simulink model "openloop_thyristor_w_control_initial_version"  (R2019b)
settings: Solver=VariableStepAuto  StartTime=0.0  StopTime=10  RelTol=1e-3
undefined symbols (not defined in the file): D1, lagging, pulse, sigbuilder_block
libraries: powerlib x20, powerlib_meascontrol x4, simulink x3
settings Model: Creator=82309  LastModifiedBy=82309
settings SolverCC: ZeroCrossAlgorithm=Adaptive
settings DebuggingCC: IgnoredZcDiagnostic=none

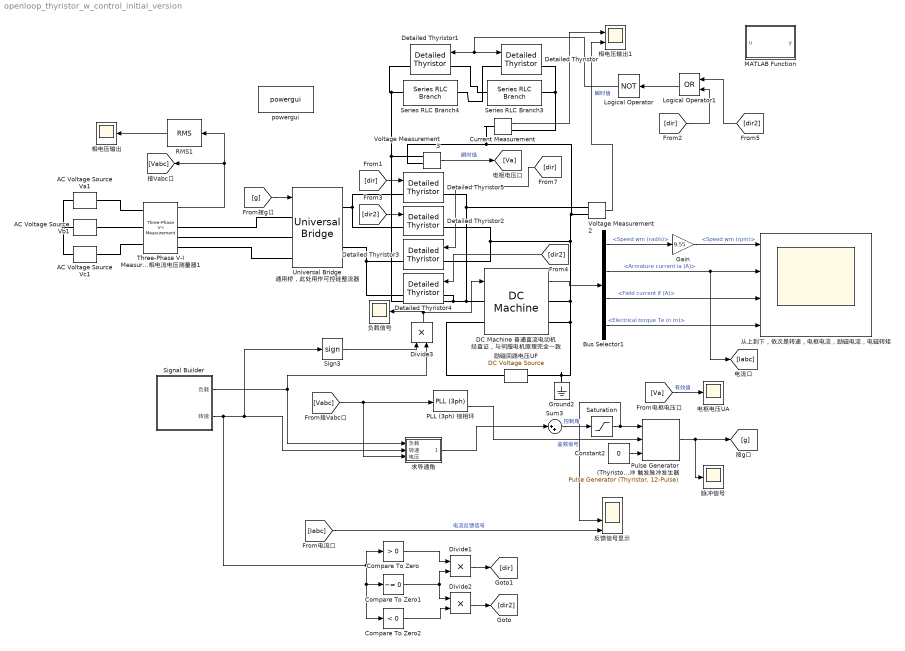
== system openloop_thyristor_w_control_initial_version ==
  AC Voltage Source Va1 : powerlib/Electrical Sources/AC Voltage Source  Amplitude=200  Phase=0  Frequency=60  SampleTime=0  Measurements=None  BusType=swing  Pref=10e3  Qref=0  Qmin=-inf  Qmax=+inf
      settings: SourceProductName=Simscape Electrical
  AC Voltage Source Vb1 : powerlib/Electrical Sources/AC Voltage Source  Amplitude=200  Phase=-120  Frequency=60  SampleTime=0  Measurements=None  BusType=swing  Pref=10e3  Qref=0  Qmin=-inf  Qmax=+inf
      settings: SourceProductName=Simscape Electrical
  AC Voltage Source Vc1 : powerlib/Electrical Sources/AC Voltage Source  Amplitude=200  Phase=-240  Frequency=60  SampleTime=0  Measurements=None  BusType=swing  Pref=10e3  Qref=0  Qmin=-inf  Qmax=+inf
      settings: SourceProductName=Simscape Electrical
  Bus Selector1 : BusSelector  OutputSignals=Speed wm (rad/s),Armature current ia (A),Field current if (A),Electrical torque Te (n m)
  Compare To Zero : simulink/Logic and Bit Operations/Compare To Zero  relop=>  OutDataTypeStr=boolean
  Compare To Zero1 : simulink/Logic and Bit Operations/Compare To Zero  relop=~=  OutDataTypeStr=boolean
  Compare To Zero2 : simulink/Logic and Bit Operations/Compare To Zero  relop=<  OutDataTypeStr=boolean
  Constant2 : Constant  Value=0
  Current Measurement : powerlib/Measurements/Current Measurement  PhasorSimulation=off  OutputType=Complex  PSBequivalent=0
      settings: SourceProductName=Simscape Electrical
  DC Machine 普通直流电动机 经查证，与伺服电机原理完全一致 : powerlib/Machines/DC Machine  PresetModel=01: 5HP 240V 1750RPM Field:300V  MechanicalLoad=Torque TL  FieldType=Wound  ShowDetailedParameters=on  MeasurementBus=off  RLa=[2.581 0.028]  RLf=[281.3 156]  Laf=0.9483  MachineConstant=Torque constant (N.m/A)  Ke=1.8  Kt=1.8  J=0.02215  Bm=0.002953  Tf=0.5161  w0=1  Ifinit=1  TsPowergui=0  TsBlock=-1
      settings: SourceProductName=Simscape Electrical
  Detailed Thyristor : powerlib/Power Electronics/Detailed Thyristor  Ron=0.001  Lon=1e-3  Vf=0.8  IL=0.1  Tq=100e-6  IC=0  Rs=inf  Cs=250e-9  Measurements=on
      settings: SourceProductName=Simscape Electrical  SourceProductBaseCode=PS
  Detailed Thyristor1 : powerlib/Power Electronics/Detailed Thyristor  Ron=0.001  Lon=1e-3  Vf=0.8  IL=0.1  Tq=100e-6  IC=0  Rs=inf  Cs=250e-9  Measurements=on
      settings: SourceProductName=Simscape Electrical  SourceProductBaseCode=PS
  Detailed Thyristor{2..5} (4 alike) : powerlib/Power Electronics/Detailed Thyristor  Ron=0.001  Lon=1e-3  Vf=0.8  IL=0.1  Tq=100e-6  IC=0  Rs=500  Cs=250e-9  Measurements=on
      settings: SourceProductName=Simscape Electrical  SourceProductBaseCode=PS
  Divide1 : Product  Inputs=**
  Divide2 : Product  Inputs=**
  Divide3 : Product  Inputs=**
  Gain : Gain  Gain=9.55
  Ground2 : powerlib/Elements/Ground  LConnTagsString=a
      settings: SourceProductName=Simscape Electrical
  Logical Operator : Logic  Operator=NOT  AllPortsSameDT=off  OutDataTypeStr=boolean
  Logical Operator1 : Logic  Operator=OR  AllPortsSameDT=off  OutDataTypeStr=boolean
  MATLAB Function : MATLAB Function  TreatAsAtomicUnit=on
  PLL (3ph) 锁相环 : powerlib_meascontrol/PLL/PLL (3ph)  Fmin=48  Par_Init=[0, 50]  ParK=[180, 3200, 1]  TcD=1e-4  MaxRateChangeFreq=12  FilterCutOffFreq=25  Ts=0  AGC=on
      settings: SourceProductName=Simscape Electrical
  "Pulse Generator (Thyristor, 6-Pulse) 六脉冲 触发脉冲发生器" : powerlib_meascontrol/Pulse & Signal Generators/Pulse Generator (Thyristor, 12-Pulse)  GenType=6-pulse  Delta=D1 (lagging)  pwidth=10  Double_Pulse=on  Ts=0
      settings: SourceProductName=Simscape Electrical  SourceProductBaseCode=PS
  RMS1 : powerlib_meascontrol/Measurements/RMS  TrueRMS=on  Freq=60  RMSInit=0  Ts=0
      settings: SourceProductName=Simscape Electrical
  Saturation : Saturate  UpperLimit=180  LowerLimit=0
  Series RLC Branch3 : powerlib/Elements/Series RLC Branch  LConnTagsString=__new0  RConnTagsString=__new0  BranchType=R  Resistance=1  Inductance=0.01  SetiL0=off  InitialCurrent=0  Capacitance=1e-6  Setx0=off  InitialVoltage=0  Measurements=None
      settings: SourceProductName=Simscape Electrical
  Series RLC Branch4 : powerlib/Elements/Series RLC Branch  LConnTagsString=__new0  RConnTagsString=__new0  BranchType=R  Resistance=1  Inductance=0.01  SetiL0=off  InitialCurrent=0  Capacitance=1e-6  Setx0=off  InitialVoltage=0  Measurements=None
      settings: SourceProductName=Simscape Electrical
  Sign3 : Signum
  Signal Builder : Subsystem  Tag=STV Subsys  LoadFcn=sigbuilder_block('load',[481.8 72 550.8 363.6 ]);  StartFcn=sigbuilder_block('start');  StopFcn=sigbuilder_block('stop');  ClipboardFcn=sigbuilder_block('clipboard');  mask(Sigbuilder block){tuvar=[0:10]}
      mask help: Sigbuilder GUI
      mask init:
      | if ~strcmp(get_param(bdroot(gcbh),'SimulationStatus'),'stopped') tuvar = sigbuilder_block('maskInit'); end
      settings: CopyFcn=sigbuilder_block('copy');  DeleteFcn=sigbuilder_block('delete');  ModelCloseFcn=sigbuilder_block('modelClose');  PreSaveFcn=sigbuilder_block('preSave');  PauseFcn=sigbuilder_block('pause')  ContinueFcn=sigbuilder_block('continue')  NameChangeFcn=sigbuilder_block('namechange');  OpenFcn=sigbuilder_block('open',[-27 31.8 550.8 363.6 ]);  CloseFcn=sigbuilder_block('close');
      mask Display: plot(0, 0, 100, 100,[2, 2, 32, 32, 2], [68, 8, 8, 68, 68],[32, 2], [38, 38], [32, 19, 2],[53, 60, 44], [32, 17, 17, 2],[16, 16, 31, 31]);txt = getActiveGroup(gcbh);text(2, 100, txt,'verticalAlignment', 'top');
  Sum3 : Sum  Inputs=|++
  Three-Phase V-I Measurement 三相电流电压测量器1 : powerlib/Measurements/Three-Phase V-I Measurement  VoltageMeasurement=phase-to-ground  SetLabelV=off  LabelV=Vabc  Vpu=off  VpuLL=off  CurrentMeasurement=yes  SetLabelI=off  LabelI=Iabc  Ipu=off  Pbase=100e6  Vbase=500e3  OutputType=Complex  PhasorSimulation=off  PSBequivalent=0
      settings: SourceProductName=Simscape Electrical
  Universal Bridge 通用桥，此处用作可控硅整流器 : powerlib/Power Electronics/Universal Bridge  Arms=3  SnubberResistance=1e5  SnubberCapacitance=inf  Device=Thyristors  Ron=1e-3  Lon=0  ForwardVoltages="[  0  0  ]"  ForwardVoltage=0  GTOparameters=[ 10e-6 , 20e-6 ]  IGBTparameters=[ 1e-6 , 2e-6 ]  Measurements=None  Measurements_2=None  converterType=Rectifier
      settings: SourceProductName=Simscape Electrical
  Voltage Measurement2 : powerlib/Measurements/Voltage Measurement  PhasorSimulation=off  OutputType=Complex  PSBequivalent=0
      settings: SourceProductName=Simscape Electrical
  Voltage Measurement3 : powerlib/Measurements/Voltage Measurement  PhasorSimulation=off  OutputType=Complex  PSBequivalent=0
      settings: SourceProductName=Simscape Electrical
  powergui : powerlib/powergui  Priority=1  SimulationMode=Continuous  SampleTime=50e-6  frequency=60  Iterations=50  frequencyindice=60  Pbase=100e6  ErrMax=1e-4  UnitsV=kV  UnitsW=MW  buscounter=0  FunctionMessages=off  echomessages=off  EnableUseOfTLC=off  CurrentSourceSwitches=off  DisableSnubberDevices=off  DisableRonSwitches=off  DisableVfSwitches=off  DisplayEquations=off  AutomaticDiscreteSolvers=off  SolverType=Tustin/Backward Euler (TBE)  Interpol=off  ExternalGateDelay=off  methode=off  Ts=100  x0status=blocks  SPID=on  SwTol=0  HookPort=off  NonlinearTolerance=1e-4  nMaxIteration=100  ContinueOnMaxIteration=off  RestoreLinks=warning  ResistiveCurrentMeasurement=off  Frange=[0:2:500]  Ylog=off  Xlog=on  ShowGrid=off  save=off  variable=ZData  structure=0  ZoomFFT=off  StartTime=0.0  cycles=1  DisplayStyle=1  fundamental=60  FreqAxis=off  MaxFrequency=1000  frequencyindicesteady=1  RmsSteady=1  display=off
      settings: SourceProductName=Simscape Electrical
  从上到下，依次是转速，电枢电流，励磁电流，电磁转矩 : Scope  NumInputPorts=4
  励磁回路电压UF : powerlib/Electrical Sources/DC Voltage Source  Amplitude=300  Measurements=None
      settings: SourceProductName=Simscape Electrical
  反馈信号显示 : Scope  NumInputPorts=4
  求导通角 : Subsystem
  电枢电压UA : Scope
  相电压输出 : Scope
  相电压输出1 : Scope  NumInputPorts=2
  脉冲信号 : Scope
  负载信号 : Scope
  wires:
  Bus Selector1/1 -> Gain/1  "<Speed wm (rad/s)>"
  Bus Selector1/3 -> 从上到下，依次是转速，电枢电流，励磁电流，电磁转矩/3  "<Field current if (A)>"
  "Pulse Generator (Thyristor, 6-Pulse) 六脉冲 触发脉冲发生器"/1 -> [g], 脉冲信号/1
  Three-Phase V-I Measurement 三相电流电压测量器1/1 -> RMS1/1, [Vabc]
  DC Machine 普通直流电动机 经查证，与伺服电机原理完全一致/1 -> Bus Selector1/1
  Constant2/1 -> "Pulse Generator (Thyristor, 6-Pulse) 六脉冲 触发脉冲发生器"/3
  [g] -> Universal Bridge 通用桥，此处用作可控硅整流器/1
  Bus Selector1/2 -> [Iabc], 从上到下，依次是转速，电枢电流，励磁电流，电磁转矩/2  "<Armature current ia (A)>"
  Gain/1 -> 从上到下，依次是转速，电枢电流，励磁电流，电磁转矩/1  "<Speed wm (rpm)>"
  Bus Selector1/4 -> 从上到下，依次是转速，电枢电流，励磁电流，电磁转矩/4  "<Electrical torque Te (n m)>"
  PLL (3ph) 锁相环/2 -> "Pulse Generator (Thyristor, 6-Pulse) 六脉冲 触发脉冲发生器"/2  "鉴频信号"
  [Vabc] -> PLL (3ph) 锁相环/1, 求导通角/3(电压)
  RMS1/1 -> 相电压输出/1
  Voltage Measurement3/1 -> [Va]  "瞬时值"
  Signal Builder/1(负载) -> 求导通角/1(负载), Divide3/2
  Logical Operator1/1 -> Logical Operator/1
  [Va] -> 电枢电压UA/1  "有效值"
  [Iabc] -> 反馈信号显示/4  "电流反馈信号"
  Saturation/1 -> "Pulse Generator (Thyristor, 6-Pulse) 六脉冲 触发脉冲发生器"/1, 反馈信号显示/3
  Sum3/1 -> Saturation/1  "控制角"
  求导通角/1(Out1) -> Sum3/1
  Voltage Measurement2/1 -> 相电压输出1/2  "瞬时值"
  Divide1/1 -> [dir]
  Compare To Zero/1 -> Divide1/1
  Compare To Zero1/1 -> Divide2/1, Divide1/2
  Compare To Zero2/1 -> Divide2/2
  Divide2/1 -> [dir2]
  [dir] -> Logical Operator1/2
  [dir2] -> Logical Operator1/1
  Logical Operator/1 -> Detailed Thyristor1/1, Detailed Thyristor/1
  Current Measurement/1 -> 相电压输出1/1
  [dir2] -> Detailed Thyristor2/1
  [dir] -> Detailed Thyristor5/1
  [dir2] -> Detailed Thyristor4/1
  [dir] -> Detailed Thyristor3/1
  Sign3/1 -> Divide3/1
  Divide3/1 -> DC Machine 普通直流电动机 经查证，与伺服电机原理完全一致/1, 负载信号/1
  Signal Builder/2(转速) -> Compare To Zero2/1, Compare To Zero1/1, Compare To Zero/1, Sign3/1, 求导通角/2(转速)
  connections:
  励磁回路电压UF/RConn1 -- DC Machine 普通直流电动机 经查证，与伺服电机原理完全一致/LConn2
  Three-Phase V-I Measurement 三相电流电压测量器1/RConn1 -- Universal Bridge 通用桥，此处用作可控硅整流器/LConn1
  Universal Bridge 通用桥，此处用作可控硅整流器/LConn2 -- Three-Phase V-I Measurement 三相电流电压测量器1/RConn2
  Three-Phase V-I Measurement 三相电流电压测量器1/RConn3 -- Universal Bridge 通用桥，此处用作可控硅整流器/LConn3
  Series RLC Branch3/RConn1 -- Detailed Thyristor1/LConn1
  Detailed Thyristor/LConn1 -- Series RLC Branch4/RConn1
  AC Voltage Source Vb1/LConn1 -- AC Voltage Source Vc1/LConn1 -- AC Voltage Source Va1/LConn1
  AC Voltage Source Va1/RConn1 -- Three-Phase V-I Measurement 三相电流电压测量器1/LConn1
  AC Voltage Source Vc1/RConn1 -- Three-Phase V-I Measurement 三相电流电压测量器1/LConn3
  AC Voltage Source Vb1/RConn1 -- Three-Phase V-I Measurement 三相电流电压测量器1/LConn2
  Current Measurement/RConn1 -- Series RLC Branch3/LConn1 -- Detailed Thyristor/RConn1
  Universal Bridge 通用桥，此处用作可控硅整流器/RConn1 -- Detailed Thyristor5/LConn1 -- Detailed Thyristor2/LConn1
  Detailed Thyristor3/RConn1 -- Detailed Thyristor4/RConn1 -- Universal Bridge 通用桥，此处用作可控硅整流器/RConn2
  Voltage Measurement3/LConn1 -- Detailed Thyristor1/RConn1 -- Series RLC Branch4/LConn1 -- Detailed Thyristor4/LConn1 -- Detailed Thyristor5/RConn1 -- Voltage Measurement2/LConn1 -- DC Machine 普通直流电动机 经查证，与伺服电机原理完全一致/LConn1
  DC Machine 普通直流电动机 经查证，与伺服电机原理完全一致/RConn2 -- Ground2/LConn1 -- 励磁回路电压UF/LConn1 -- Current Measurement/LConn1 -- Voltage Measurement3/LConn2 -- Voltage Measurement2/LConn2 -- Detailed Thyristor2/RConn1 -- Detailed Thyristor3/LConn1 -- DC Machine 普通直流电动机 经查证，与伺服电机原理完全一致/RConn1

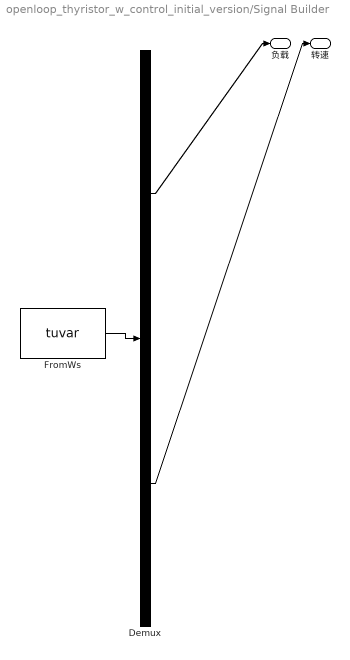
== system openloop_thyristor_w_control_initial_version/Signal Builder ==
  Demux : Demux  Tag=STV Demux  Outputs=2
  FromWs : FromWorkspace  Tag=STV FromWs  VariableName=tuvar  SampleTime=0
      SigBuilderData=|
      | common.afterFinalStr = 'Extrapolate'
      | common.sampleTime = 0
      | dataSet.timeRange = [0 10]
      | dataSet.name = 'Group 1'
      | sbobj.Groups.Name = 'Group 1'
      | sbobj.Groups.Signals(1).Name = '负载'
      | sbobj.Groups.Signals(1).XData = [0 2.44 2.44 3.58 3.58 10]
      | sbobj.Groups.Signals(1).YData = [10.3 10.3 4.6 4.6 10.2 10.2]
      | sbobj.Groups.Signals(2).Name = '转速'
      | sbobj.Groups.Signals(2).XData = [0 0.98 0.98 2.12 2.12 7.38 7.38 10]
      | sbobj.Groups.Signals(2).YData = [660 660 -150 -150 260 260 0 0]
  负载 : Outport  Tag=STV Outport
  转速 : Outport  Tag=STV Outport  Port=2
  wires:
  FromWs/1 -> Demux/1
  Demux/1 -> 负载/1
  Demux/2 -> 转速/1

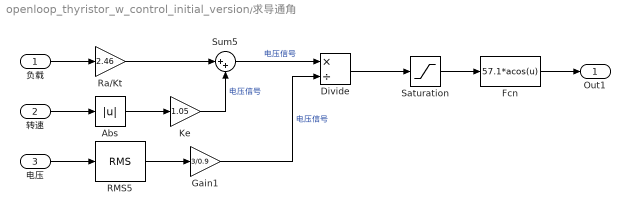
== system openloop_thyristor_w_control_initial_version/求导通角 ==
  负载 : Inport
  转速 : Inport  Port=2
  电压 : Inport  Port=3
  Abs : Abs
  Divide : Product  Inputs=*/
  Fcn : Fcn  Expr=57.1*acos(u)
  Gain1 : Gain  Gain=3/0.9
  "Ke " : Gain  Gain=1.05
  RMS5 : powerlib_meascontrol/Measurements/RMS  TrueRMS=on  Freq=60  RMSInit=0  Ts=0
      settings: SourceProductName=Simscape Electrical
  Ra/Kt : Gain  Gain=2.46
  Saturation : Saturate  UpperLimit=1  LowerLimit=-1
  Sum5 : Sum  Inputs=|++
  Out1 : Outport
  wires:
  "Ke "/1 -> Sum5/2  "电压信号"
  负载/1 -> Ra/Kt/1
  Sum5/1 -> Divide/1  "电压信号"
  Divide/1 -> Saturation/1
  转速/1 -> Abs/1
  Abs/1 -> "Ke "/1
  电压/1 -> RMS5/1
  Ra/Kt/1 -> Sum5/1
  RMS5/1 -> Gain1/1
  Fcn/1 -> Out1/1
  Saturation/1 -> Fcn/1
  Gain1/1 -> Divide/2  "电压信号"

== matlab function openloop_thyristor_w_control_initial_version/MATLAB Function ==
  data: u input; y output
function y = fcn(u)
if u>30
    y=0;
else
    y=1;
end
